simulink model "sdrzQPSKRxFPGAretarget"  (R2016a)
settings: Solver=FixedStepDiscrete  SolverMode=SingleTasking  StartTime=0.0  StopTime=inf  RelTol=1e-3
PreLoadFcn:
  | sdrzQPSKRxFPGAretarget_params = sdrzQPSKRxFPGA_init;
InitFcn:
  | sdrzQPSKRxFPGAretarget_params = sdrzQPSKRxFPGA_init;
libraries: hdlsllib x3, sdrzblksprivate x1, commsequence2 x1, sdrzlib x1
CloseFcn:
  | clear sdrzQPSKRxFPGAretarget_params;
Description:
  | This model uses a targeted .bit generated from the sdrzQPSKRxFPGA example to receive a QPSK signal using SDR hardware
settings Model: FPTRunName=Active  ModifiedByFormat=The MathWorks Inc.  SimulationMode=accelerator  Creator=The MathWorks, Inc.  LastModifiedBy=The MathWorks Inc.
settings DataIOCC: LimitDataPoints=on  SaveFormat=Structure  SaveOutput=off  SignalLogging=off  DSMLogging=off  SaveTime=off
settings OptimizationCC: BlockReduction=off  ConditionallyExecuteInputs=off  DefaultParameterBehavior=Inlined  ExpressionDepthLimit=2147483647  LocalBlockOutputs=off  SimCompilerOptimization=on
settings DebuggingCC: AlgebraicLoopMsg=error  UnderspecifiedInitializationDetection=Classic  MergeDetectMultiDrivingBlocksExec=none  SolverPrmCheckMsg=warning  MultiTaskDSMMsg=warning  MultiTaskCondExecSysMsg=none  SingleTaskRateTransMsg=error  ParameterPrecisionLossMsg=none  FcnCallInpInsideContextMsg=UseLocalSettings  AllowSymbolicDim=off  StateNameClashWarn=warning
settings HardwareCC: ProdBitPerPointer=32  ProdLargestAtomicFloat=None  ProdIntDivRoundTo=Undefined  ProdEndianess=Unspecified  ProdWordSize=32  ProdHWDeviceType=ASIC/FPGA->ASIC/FPGA  TargetBitPerPointer=64  TargetLongLongMode=on  TargetIntDivRoundTo=Zero  TargetEndianess=LittleEndian  TargetWordSize=64  TargetHWDeviceType=MATLAB Host  ProdEqTarget=off
settings ModelReferenceCC: PropagateSignalLabelsOutOfModel=off
settings RTWCC: CustomSourceCode=|
  | #include <stdio.h>
  | #include <stdlib.h>
settings GRTTargetCC: CombineOutputUpdateFcns=off  GRTInterface=on
settings ConfigComp: CovModelRefEnable=Off  CovSFcnEnable=off

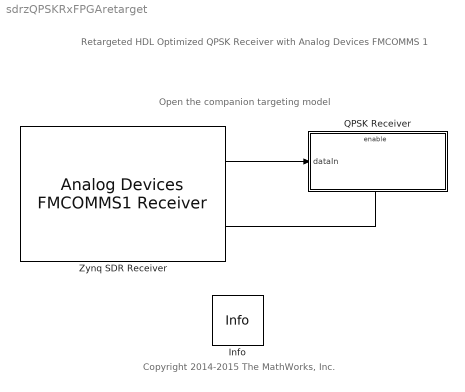
== system sdrzQPSKRxFPGAretarget ==
  note: Copyright 2014-2015 The MathWorks, Inc.
  note: Retargeted HDL Optimized QPSK Receiver
      | with Analog Devices FMCOMMS 1
  note: Open the companion targeting model
  Info : sdrzblksprivate/Info  SystemSampleTime=-1
  QPSK Receiver : Subsystem
      mask Display: disp('QPSK Receiver')
  Zynq SDR Receiver : sdrzlib/Analog Devices FMCOMMS1 Receiver  SourceLibraryInfo="This block requires Communications System Toolbox Support Package for Xilinx FPGA-Based Radio. <a href=\"http://www.mathworks.com/hardware-support-packages\">More information</a>"  sobjType=comm.SDRZynqFMCOMMS1Receiver  IPAddress=192.168.3.2  dataUDPPort=-1  ctrlUDPPort=-1  subDeviceList=comm.SDRZynqFMCOMMS1Receiver  sdrBlockType=SDRBlockTypeSLT.SDRRxBlock  requester=UNUSED_BY_SFCN  sdrExecutionMode=HW  LostSamplesOutputPort=off  OutputDataType=int16  FrameLength=sdrzQPSKRxFPGAretarget_params.Upsampling*sdrzQPSKRxFPGAretarget_params.FrameSize*sdrzQPSKRxFPGAretarget_params.RxBufferedFrames  EnableBurstMode=off  NumFramesInBurst=500  BypassUserLogic=off  DecimatorSelect=DDC decimator  SourceSelect=RF data  SineAmplitude=16000  SineFrequency=30000  EnableInternalClock=off  BypassIQBalance=on  CenterFrequencySource=Dialog  CenterFrequency=sdrzQPSKRxFPGAretarget_params.RadioCenterFrequency  IntermediateFrequencySource=Dialog  IntermediateFrequency=sdrzQPSKRxFPGAretarget_params.RadioIntermediateFrequency  IFBandwidthSource=Dialog  IFBandwidth=40e6  ADCRateSource=Dialog  ADCRate=sdrzQPSKRxFPGAretarget_params.RadioADCRate  GainSource=Dialog  Gain=sdrzQPSKRxFPGAretarget_params.RadioGain  DecimationFactorSource=Dialog  DecimationFactor=sdrzQPSKRxFPGAretarget_params.RadioDecimationFactor  RFFrequencyIsTunable=logical(0)  SampleTime=sdrzQPSKRxFPGAretarget_params.Ts  BypassDCBlockingFilter=off  IQBalanceCoefficients=64  SkipAllHardwareResetAndInitialization=off  EnableIQCalibrationTable=on  CacheIQCalibrationTable=off
  wires:
  Zynq SDR Receiver/1 -> QPSK Receiver/1(dataIn)
  Zynq SDR Receiver/2 -> QPSK Receiver/Enable

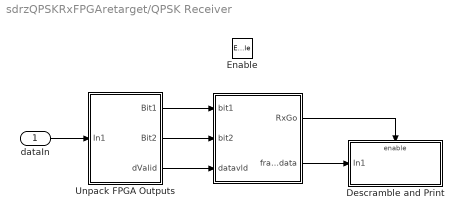
== system sdrzQPSKRxFPGAretarget/QPSK Receiver ==
  dataIn : Inport  OutDataTypeStr=int16
  Enable : EnablePort
  " " : MATLAB Function  TreatAsAtomicUnit=on
  Descramble and Print : Subsystem  TreatAsAtomicUnit=on
  Unpack FPGA Outputs : Subsystem
  wires:
  Unpack FPGA Outputs/2(Bit2) -> " "/2(bit2)
  Unpack FPGA Outputs/1(Bit1) -> " "/1(bit1)
  Unpack FPGA Outputs/3(dValid) -> " "/3(datavld)
  dataIn/1 -> Unpack FPGA Outputs/1(In1)
  " "/1(RxGo) -> Descramble and Print/Enable
  " "/2(framed_data) -> Descramble and Print/1(In1)

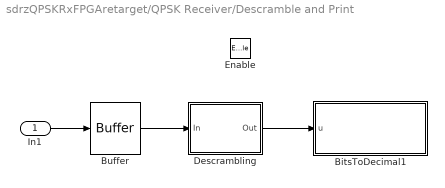
== system sdrzQPSKRxFPGAretarget/QPSK Receiver/Descramble and Print ==
  In1 : Inport
  Enable : EnablePort
  BitsToDecimal1 : MATLAB Function  TreatAsAtomicUnit=on
  Buffer : Buffer  N=200  TreatMby1Signals=One channel  OutputFrames=off
  Descrambling : Subsystem
      mask Display: disp('Descrambling')
  wires:
  Descrambling/1(Out) -> BitsToDecimal1/1(u)
  In1/1 -> Buffer/1
  Buffer/1 -> Descrambling/1(In)

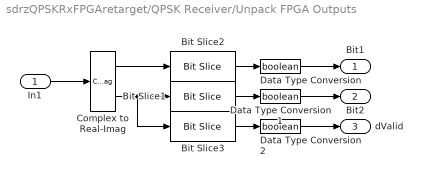
== system sdrzQPSKRxFPGAretarget/QPSK Receiver/Unpack FPGA Outputs ==
  In1 : Inport
  Bit Slice1 : hdlsllib/HDL Operations/Bit Slice  lidx=0  ridx=0
  Bit Slice2 : hdlsllib/HDL Operations/Bit Slice  lidx=0  ridx=0
  Bit Slice3 : hdlsllib/HDL Operations/Bit Slice  lidx=15  ridx=15
  Complex to Real-Imag : ComplexToRealImag
  Data Type Conversion : DataTypeConversion  OutDataTypeStr=boolean
  Data Type Conversion1 : DataTypeConversion  OutDataTypeStr=boolean
  Data Type Conversion2 : DataTypeConversion  OutDataTypeStr=boolean
  Bit1 : Outport
  Bit2 : Outport  Port=2
  dValid : Outport  Port=3
  wires:
  In1/1 -> Complex to Real-Imag/1
  Complex to Real-Imag/1 -> Bit Slice2/1
  Complex to Real-Imag/2 -> Bit Slice3/1, Bit Slice1/1
  Bit Slice2/1 -> Data Type Conversion/1
  Bit Slice1/1 -> Data Type Conversion1/1
  Bit Slice3/1 -> Data Type Conversion2/1
  Data Type Conversion/1 -> Bit1/1
  Data Type Conversion1/1 -> Bit2/1
  Data Type Conversion2/1 -> dValid/1

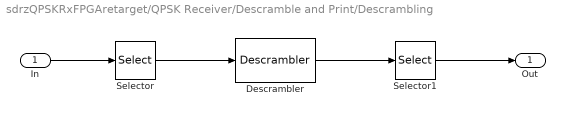
== system sdrzQPSKRxFPGAretarget/QPSK Receiver/Descramble and Print/Descrambling ==
  In : Inport
  Descrambler : commsequence2/Descrambler  M=2  poly=[1 1 1 0 1]  iniStaSource=Dialog Parameter  ini_sta=[0 0 0 0]  resetViaPort=off
  Selector : Selector  IndexOptions=Index vector (dialog)  Indices=[sdrzQPSKRxFPGAretarget_params.BarkerLength*log2(sdrzQPSKRxFPGAretarget_params.M)+1:sdrzQPSKRxFPGAretarget_params.FrameSize*log2(sdrzQPSKRxFPGAretarget_params.M)]  OutputSizes=1
  Selector1 : Selector  IndexOptions=Index vector (dialog)  Indices=[1:sdrzQPSKRxFPGAretarget_params.MsgLength]  OutputSizes=1
  Out : Outport
  wires:
  Descrambler/1 -> Selector1/1
  Selector1/1 -> Out/1
  In/1 -> Selector/1
  Selector/1 -> Descrambler/1

== matlab function sdrzQPSKRxFPGAretarget/QPSK Receiver/  ==
  data: RxGo output; framed_data output; bit1 input; bit2 input; datavld input
function [RxGo, framed_data] = dataframer(bit1, bit2, datavld)
%#codegen

persistent  gooddata_from_prev length_prev_good_data


if isempty(gooddata_from_prev)
    gooddata_from_prev = false(8000,1);
    length_prev_good_data = 0;
end

gooddata_current = false(8000,1); % worst case scenario
if any(datavld) % there is some valid data
    % get the valid data from this frame and append it with the previous
    % stored one, if any
    
    %gooddata_current = false(2*sum(datavld),1);
    gooddata_current(1:2:2*sum(datavld)-1) = bit1(logical(datavld));
    gooddata_current(2:2:2*sum(datavld))   = bit2(logical(datavld));
    % append with prev good data
    data_tmp = [gooddata_from_prev(1:length_prev_good_data);gooddata_current(1:2*sum(datavld))];
    if length(data_tmp) > 8000
        framed_data = data_tmp(1:8000);
        RxGo = 1;
        gooddata_length_athand = length(data_tmp);
        datalen_fornext = gooddata_length_athand -8000;
        gooddata_from_prev(1:datalen_fornext) = data_tmp(8001:8001+datalen_fornext-1);
        length_prev_good_data = datalen_fornext;
    elseif length(data_tmp) == 8000
        framed_data = data_tmp(1:8000);
        RxGo = 1;
        gooddata_from_prev =  false(8000,1);
        length_prev_good_data = 0;
    else % less than 8000
        gooddata_length_athand = length(data_tmp);
        datalen_fornext = gooddata_length_athand;      
        gooddata_from_prev(1:gooddata_length_athand) = data_tmp(1:gooddata_length_athand);
        length_prev_good_data = datalen_fornext;
        framed_data = false(8000,1); % garbage
        RxGo = 0;
    end
    
else % none of the data is valid
    RxGo = 0;
    framed_data = false(8000,1); %just send the data through
    gooddata_from_prev = false(8000,1);
    length_prev_good_data = 0;
end

== matlab function sdrzQPSKRxFPGAretarget/QPSK Receiver/Descramble and Print/BitsToDecimal1 ==
  data: u input
function BitsToASCII(u)
% Convert bits to ASCII message.

persistent package_counter;
persistent error_counter;
if isempty(package_counter)
    package_counter = 0;
    error_counter   = 0;
end

coder.extrinsic('disp')
coder.extrinsic('num2str')

aa = de2bi(int8('Hello world 0'),7,'left-msb');
bits_ref = double(reshape(aa.',1,[]));
bits_ref = bits_ref(:);

error_counter   = error_counter   + sum(abs(bits_ref - u(1:91)));
package_counter = package_counter + 1;

% Convert binary-valued column vector to 7-bit decimal values.
w = [64 32 16 8 4 2 1]; % binary digit weighting
Nbits = numel(u);
Ny = Nbits/7;
y = zeros(1,Ny);
for i = 0:Ny-1
    y(i+1) = w*u(7*i+(1:7));
end

% Display ASCII message to command window
disp(char(y));
